simulink model "ASSIG2_v3"  (R2020a)
settings: Solver=FixedStepAuto  StartTime=0.0  StopTime=10.0  FixedStep=1e-3  RelTol=1e-3  EnableMultiTasking=on
undefined symbols (not defined in the file): A0, A1, D0, D1, D10, D11, D12, D13, D2, D3, D4, D5, D6, D7, D8, D9, magnitude, PTA0, PTA1, PTA2, PTB2, PTB23, PTB3, PTB9, PTC16, PTC17, PTC2, PTC3, PTC4, PTD0, PTD1, PTD2, PTD3
libraries: frdmk64flib x19, etargetslib x2
settings Model: ExtModeTrigDuration=5  Creator=Nour  LastModifiedBy=Khaled
settings OptimizationCC: EnhancedBackFolding=on  PassReuseOutputArgsAs=Individual arguments  ZeroExternalMemoryAtStartup=off  ZeroInternalMemoryAtStartup=off  MaxStackSize=64  OptimizeBlockOrder=speed  DifferentSizesBufferReuse=on  OptimizationCustomize=off  EfficientTunableParamExpr=on
settings DebuggingCC: ParameterTunabilityLossMsg=error
settings HardwareCC: ProdBitPerPointer=32  ProdBitPerSizeT=32  ProdBitPerPtrDiffT=32  ProdLargestAtomicInteger=Long  ProdLargestAtomicFloat=Double  ProdWordSize=32  ProdHWDeviceType=ARM Compatible->ARM Cortex
settings SFSimCC: MATLABDynamicMemAlloc=off
settings RTWCC: SystemTargetFile=ert.tlc  HardwareBoard=NXP FRDM-K64F  TemplateMakefile=ert_default_tmf  Toolchain=GNU Tools for ARM Embedded Processors
settings CodeAppCC: ForceParamTrailComments=on  IgnoreCustomStorageClasses=off  OperatorAnnotations=on  SimulinkDataObjDesc=on  SFDataObjDesc=on  InsertBlockDesc=on

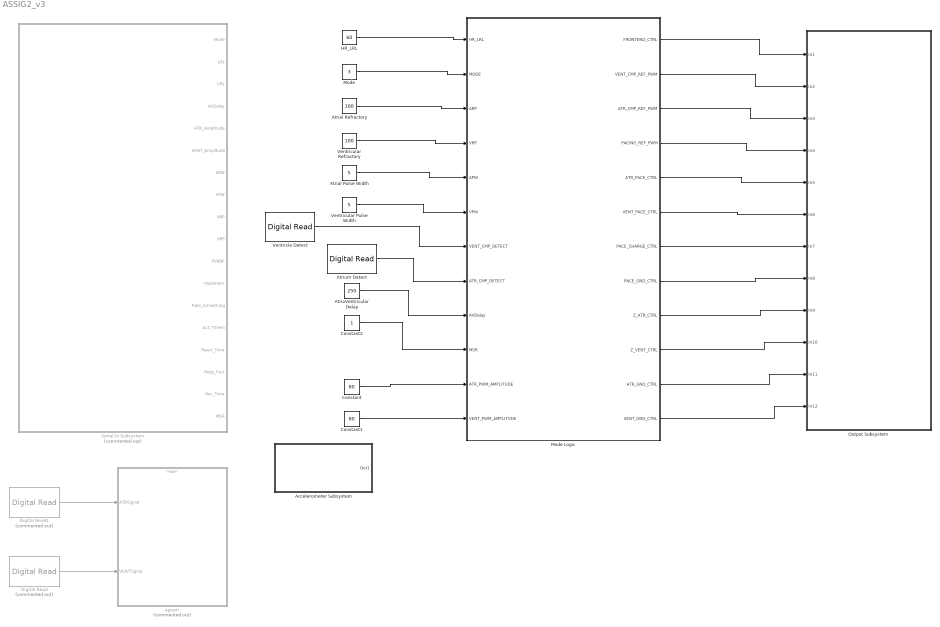
== system ASSIG2_v3 ==
  Accelerometer Subsystem : Subsystem
  Atrial Pulse Width : Constant  Value=5  OutDataTypeStr=uint16
  Atrial Refractory : Constant  Value=100  OutDataTypeStr=uint16
  AtrioVentricular Delay : Constant  Value=250  OutDataTypeStr=uint16
  Atrium Detect : frdmk64flib/Digital Read  Whichpin=PTC16 (D0)  SampleTime=-1
  Constant : Constant  Value=80  OutDataTypeStr=uint16
  Constant1 : Constant  Value=80  OutDataTypeStr=uint16
  Constant2 : Constant  OutDataTypeStr=uint16
  Digital Read : frdmk64flib/Digital Read  Commented=on  Whichpin=PTB3 (A1)  SampleTime=-1
  Digital Read1 : frdmk64flib/Digital Read  Commented=on  Whichpin=PTB2 (A0)  SampleTime=-1
  HR_LRL : Constant  Value=60  OutDataTypeStr=uint16
  Mode : Constant  Value=3  OutDataTypeStr=uint16
  Mode Logic : Stateflow chart  TreatAsAtomicUnit=on
  Output Subsystem : Subsystem
  Serial In Subsystem : Subsystem  Commented=on
  Ventricle Detect : frdmk64flib/Digital Read  Whichpin=PTC17 (D1)  SampleTime=-1
  Ventricular Pulse Width : Constant  Value=5  OutDataTypeStr=uint16
  Ventricular Refractory : Constant  Value=100  OutDataTypeStr=uint16
  egram : Subsystem  Commented=on
  wires:
  HR_LRL/1 -> Mode Logic/1(HR_LRL)
  Mode/1 -> Mode Logic/2(MODE)
  Atrial Refractory/1 -> Mode Logic/3(ARP)
  Ventricular Refractory/1 -> Mode Logic/4(VRP)
  Atrial Pulse Width/1 -> Mode Logic/5(APW)
  Ventricle Detect/1 -> Mode Logic/7(VENT_CMP_DETECT)
  Atrium Detect/1 -> Mode Logic/8(ATR_CMP_DETECT)
  Ventricular Pulse Width/1 -> Mode Logic/6(VPW)
  AtrioVentricular Delay/1 -> Mode Logic/9(AVDelay)
  Constant2/1 -> Mode Logic/10(MSR)
  Constant/1 -> Mode Logic/11(ATR_PWM_AMPLITUDE)
  Constant1/1 -> Mode Logic/12(VENT_PWM_AMPLITUDE)
  Mode Logic/1(FRONTEND_CTRL) -> Output Subsystem/1(In1)
  Mode Logic/2(VENT_CMP_REF_PWM) -> Output Subsystem/2(In2)
  Mode Logic/3(ATR_CMP_REF_PWM) -> Output Subsystem/3(In3)
  Mode Logic/4(PACING_REF_PWM) -> Output Subsystem/4(In4)
  Mode Logic/5(ATR_PACE_CTRL) -> Output Subsystem/5(In5)
  Mode Logic/6(VENT_PACE_CTRL) -> Output Subsystem/6(In6)
  Mode Logic/7(PACE_CHARGE_CTRL) -> Output Subsystem/7(In7)
  Mode Logic/8(PACE_GND_CTRL) -> Output Subsystem/8(In8)
  Mode Logic/9(Z_ATR_CTRL) -> Output Subsystem/9(In9)
  Mode Logic/10(Z_VENT_CTRL) -> Output Subsystem/10(In10)
  Mode Logic/11(ATR_GND_CTRL) -> Output Subsystem/11(In11)
  Mode Logic/12(VENT_GND_CTRL) -> Output Subsystem/12(In12)
  Digital Read/1 -> egram/2(VENTSignal)
  Digital Read1/1 -> egram/1(ATRSignal)

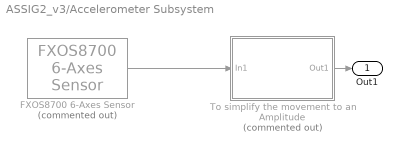
== system ASSIG2_v3/Accelerometer Subsystem ==
  FXOS8700 6-Axes Sensor : frdmk64flib/FXOS8700 6-Axes Sensor  Commented=on  Activesensor=Accelerometer only  ODR=800Hz  HybridODR=400Hz  Accelfullrange=-4g to +4g  SampleTime=-1
  To simplify the movement to an Amplitude : Subsystem  Commented=on
  Out1 : Outport
  wires:
  FXOS8700 6-Axes Sensor/1 -> To simplify the movement to an Amplitude/1(In1)
  To simplify the movement to an Amplitude/1(Out1) -> Out1/1

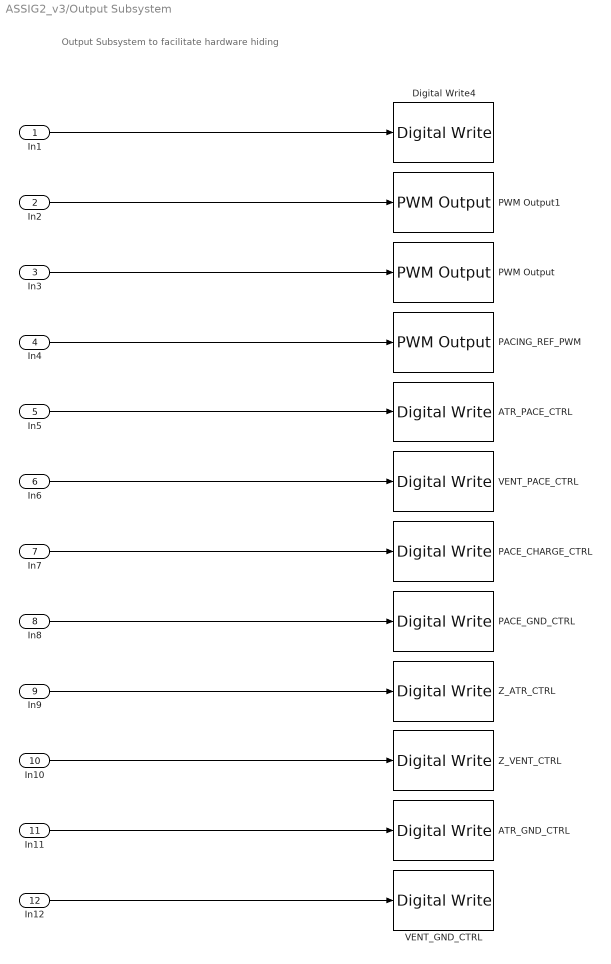
== system ASSIG2_v3/Output Subsystem ==
  note: Output Subsystem to facilitate hardware hiding
  In1 : Inport
  In2 : Inport  Port=2
  In3 : Inport  Port=3
  In4 : Inport  Port=4
  In5 : Inport  Port=5
  In6 : Inport  Port=6
  In7 : Inport  Port=7
  In8 : Inport  Port=8
  In9 : Inport  Port=9
  In10 : Inport  Port=10
  In11 : Inport  Port=11
  In12 : Inport  Port=12
  ATR_GND_CTRL : frdmk64flib/Digital Write  Whichpin=PTD2 (D11)
  ATR_PACE_CTRL : frdmk64flib/Digital Write  Whichpin=PTA0 (D8)
  Digital Write4 : frdmk64flib/Digital Write  Whichpin=PTD1 (D13)
  PACE_CHARGE_CTRL : frdmk64flib/Digital Write  Whichpin=PTB9 (D2)
  PACE_GND_CTRL : frdmk64flib/Digital Write  Whichpin=PTD0 (D10)
  PACING_REF_PWM : frdmk64flib/PWM Output  Whichpin=PTA2 (D5)  InitialFrequency=2000  InitialDutyCycle=80
  PWM Output : frdmk64flib/PWM Output  Whichpin=PTC2 (D6)  InitialFrequency=2000  InitialDutyCycle=20
  PWM Output1 : frdmk64flib/PWM Output  Whichpin=PTA1 (D3)  InitialFrequency=2000  InitialDutyCycle=20
  VENT_GND_CTRL : frdmk64flib/Digital Write  Whichpin=PTD3 (D12)
  VENT_PACE_CTRL : frdmk64flib/Digital Write  Whichpin=PTC4 (D9)
  Z_ATR_CTRL : frdmk64flib/Digital Write  Whichpin=PTB23 (D4)
  Z_VENT_CTRL : frdmk64flib/Digital Write  Whichpin=PTC3 (D7)
  wires:
  In7/1 -> PACE_CHARGE_CTRL/1
  In12/1 -> VENT_GND_CTRL/1
  In1/1 -> Digital Write4/1
  In4/1 -> PACING_REF_PWM/1
  In8/1 -> PACE_GND_CTRL/1
  In6/1 -> VENT_PACE_CTRL/1
  In9/1 -> Z_ATR_CTRL/1
  In10/1 -> Z_VENT_CTRL/1
  In11/1 -> ATR_GND_CTRL/1
  In2/1 -> PWM Output1/1
  In5/1 -> ATR_PACE_CTRL/1
  In3/1 -> PWM Output/1

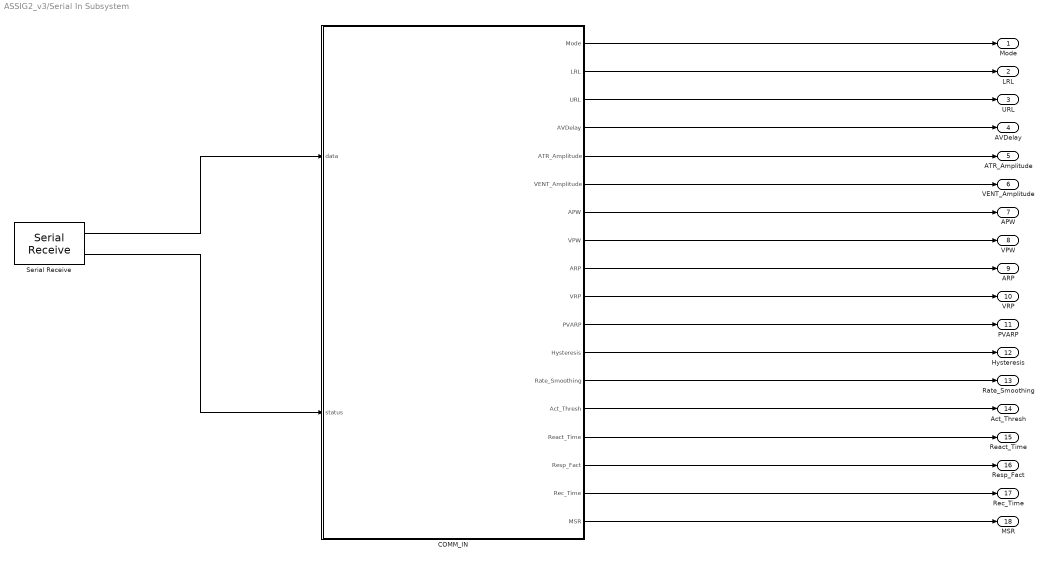
== system ASSIG2_v3/Serial In Subsystem ==
  COMM_IN : Stateflow chart  TreatAsAtomicUnit=on
  Serial Receive : frdmk64flib/Serial Receive  SCIModule=0  Baudrate=uint32(9600)  Parity=None  StopBits=1  HardwareFlowControl=None  ByteOrder=LittleEndian  DataType=uint8  DataLength=24  BlockingMode=off  OutputStatus=on  SampleTime=-1
  Mode : Outport
  LRL : Outport  Port=2
  URL : Outport  Port=3
  AVDelay : Outport  Port=4
  ATR_Amplitude : Outport  Port=5
  VENT_Amplitude : Outport  Port=6
  APW : Outport  Port=7
  VPW : Outport  Port=8
  ARP : Outport  Port=9
  VRP : Outport  Port=10
  PVARP : Outport  Port=11
  Hysteresis : Outport  Port=12
  Rate_Smoothing : Outport  Port=13
  Act_Thresh : Outport  Port=14
  React_Time : Outport  Port=15
  Resp_Fact : Outport  Port=16
  Rec_Time : Outport  Port=17
  MSR : Outport  Port=18
  wires:
  COMM_IN/3(URL) -> URL/1
  COMM_IN/9(ARP) -> ARP/1
  COMM_IN/4(AVDelay) -> AVDelay/1
  Serial Receive/1 -> COMM_IN/1(data)
  COMM_IN/2(LRL) -> LRL/1
  COMM_IN/8(VPW) -> VPW/1
  Serial Receive/2 -> COMM_IN/2(status)
  COMM_IN/6(VENT_Amplitude) -> VENT_Amplitude/1
  COMM_IN/5(ATR_Amplitude) -> ATR_Amplitude/1
  COMM_IN/16(Resp_Fact) -> Resp_Fact/1
  COMM_IN/1(Mode) -> Mode/1
  COMM_IN/13(Rate_Smoothing) -> Rate_Smoothing/1
  COMM_IN/15(React_Time) -> React_Time/1
  COMM_IN/10(VRP) -> VRP/1
  COMM_IN/7(APW) -> APW/1
  COMM_IN/17(Rec_Time) -> Rec_Time/1
  COMM_IN/18(MSR) -> MSR/1
  COMM_IN/12(Hysteresis) -> Hysteresis/1
  COMM_IN/14(Act_Thresh) -> Act_Thresh/1
  COMM_IN/11(PVARP) -> PVARP/1

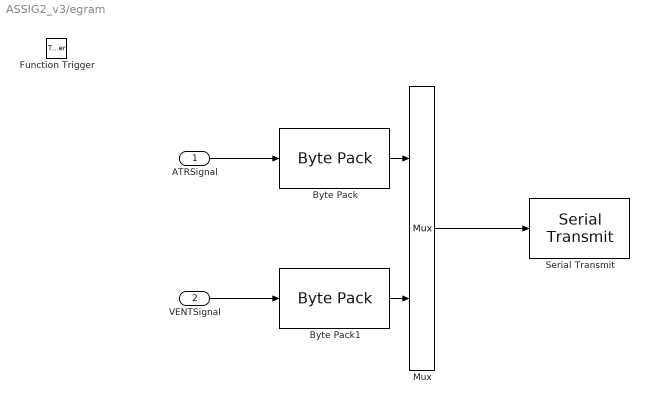
== system ASSIG2_v3/egram ==
  ATRSignal : Inport
  VENTSignal : Inport  Port=2
  Function Trigger : TriggerPort  TriggerType=function-call  IsSimulinkFunction=on  FunctionName=send_params  VariantControl=Variant  PortDimensions=1
  Byte Pack : etargetslib/Byte Pack  datatypes={'double'}  byteAlign=1
  Byte Pack1 : etargetslib/Byte Pack  datatypes={'double'}  byteAlign=1
  Mux : Mux  Inputs=2
  Serial Transmit : frdmk64flib/Serial Transmit  SCIModule=0  Baudrate=uint32(9600)  Parity=None  StopBits=1  HardwareFlowControl=None  ByteOrder=LittleEndian  BlockingMode=on  OutputStatus=off
  wires:
  ATRSignal/1 -> Byte Pack/1
  Byte Pack1/1 -> Mux/2
  Byte Pack/1 -> Mux/1
  VENTSignal/1 -> Byte Pack1/1
  Mux/1 -> Serial Transmit/1

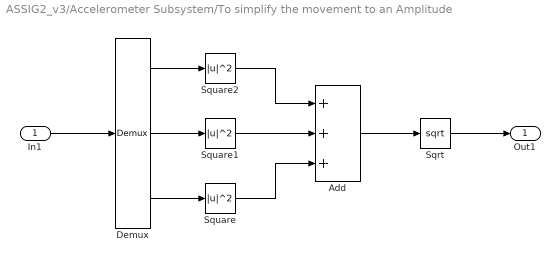
== system ASSIG2_v3/Accelerometer Subsystem/To simplify the movement to an Amplitude ==
  In1 : Inport
  Add : Sum  Inputs=+++
  Demux : Demux  Outputs=3
  Sqrt : Sqrt  OutputSignalType=real  OutDataTypeStr=uint16  SaturateOnIntegerOverflow=on
  Square : Math  Operator=magnitude^2  SaturateOnIntegerOverflow=on
  Square1 : Math  Operator=magnitude^2  SaturateOnIntegerOverflow=on
  Square2 : Math  Operator=magnitude^2  SaturateOnIntegerOverflow=on
  Out1 : Outport
  wires:
  In1/1 -> Demux/1
  Demux/3 -> Square/1
  Demux/2 -> Square1/1
  Demux/1 -> Square2/1
  Square2/1 -> Add/1
  Square1/1 -> Add/2
  Square/1 -> Add/3
  Add/1 -> Sqrt/1
  Sqrt/1 -> Out1/1

== stateflow chart ASSIG2_v3/Serial In Subsystem/COMM_IN ==
  state SET_PARAM
    %% setting parameter values through
    %% serial communication
    Mode = typecast(data(3), 'uint8');
    URL = typecast(data(4), 'uint8');
    LRL = typecast(data(5), 'uint8');
    VENT_Amplitude = typecast(data(6), 'uint8');
    VPW = typecast(data(7), 'uint8');
    ATR_Amplitude = typecast(data(8), 'uint8');
    APW = typecast(data(9), 'uint8');
    VRP = typecast(data(10:11), 'uint16');
    ARP = typecast(data(12:13), 'uint16');
    PVARP = typecast(data(14:15), 'uint16');
    Hysteresis = typecast(data(16), 'uint8');
    Rate_Smoothing = typecast(data(17), 'uint8');
    AVDelay = typecast(data(18: 19), 'uint16');
    MSR = typecast(data(20), 'uint8');
    Act_Thresh = typecast(data(21), 'uint8');
    React_Time = typecast(data(22), 'uint8');
    Resp_Fact = typecast(data(23), 'uint8');
    Rec_Time = typecast(data(24), 'uint8');
  state INITIAL
    %% Setting initial, default values of parameters
    entry:
    Mode = 0;
    URL = 0;
    LRL = 0;
    VENT_Amplitude = 0;
    VPW = 0;
    ATR_Amplitude = 0;
    APW = 0;
    VRP = 0;
    ARP = 0;
    PVARP = 0;
    Hysteresis = 0;
    Rate_Smoothing = 0;
    AVDelay = 0;
    MSR = 0;
    Act_Thresh = 0;
    React_Time = 0;
    Resp_Fact = 0;
    Rec_Time = 0;
  state STANDBY
    %% Waiting for COM
  state ECHO_PARAM
    entry:
    %%send_params();
    %% returnparams();
  (junction 15) -> SET_PARAM [order 2] : [data(2) == hex2dec('55')]
  SET_PARAM -> STANDBY
  (default) -> INITIAL
  (junction 13) -> STANDBY [order 2]
  INITIAL -> STANDBY
  STANDBY -> (junction 13) : [status == 0]
  (junction 13) -> (junction 15) [order 1] : [data(1) == hex2dec('16')]
  (junction 15) -> ECHO_PARAM [order 1] : [data(2) == hex2dec('22')]
  ECHO_PARAM -> STANDBY
  data: data input uint8 size=[24;1]; status input uint8 size=[1;1]; Mode output uint8; LRL output uint8; URL output uint8; AVDelay output uint16; ATR_Amplitude output uint8; VENT_Amplitude output uint8; APW output uint8; VPW output uint8; ARP output uint16; VRP output uint16; PVARP output uint16; Hysteresis output uint8; Rate_Smoothing output uint8; Act_Thresh output uint8; React_Time output uint8; Resp_Fact output uint8; Rec_Time output uint8; MSR output uint8

== stateflow chart ASSIG2_v3/Mode Logic ==
  state AOOR [commented out]
  state VOOR [commented out]
  state DOOR [commented out]
  state Entry
    %% MODE Values:
    %% 1: AOO
    %% 2: VOO
    %% 3: AAI
    %% 4: VVI
    %% 5: DOO
    %% 6: AOOR
    %% 7: VOOR
    %% 8: AAIR
    %% 9:  VVIR
    %% 10: DOOR
    entry:
    ATR_CMP_REF_PWM = 80;
    VENT_CMP_REF_PWM = 20;
    %% FRONTEND_CTRL = false;
    delay = 0;
  state AAI
    state Charge
      entry:
      ATR_PACE_CTRL = false;
      VENT_PACE_CTRL = false;
      PACING_REF_PWM = ATR_PWM_AMPLITUDE;
      PACE_CHARGE_CTRL = true;
      %Discharging Blocking Capacitor
      PACE_GND_CTRL = true;
      VENT_PACE_CTRL = false;
      Z_ATR_CTRL = false;
      Z_VENT_CTRL = false;
      %% ATR_PACE_CTRL = false;
      ATR_GND_CTRL = true;
      VENT_GND_CTRL = false;FRONTEND_CTRL = true;
    state Pace
      entry:
      PACE_CHARGE_CTRL = false;
      PACE_GND_CTRL = true;
      ATR_PACE_CTRL = true;
      ATR_GND_CTRL = false;
      Z_ATR_CTRL = false;
      Z_VENT_CTRL = false;
      VENT_GND_CTRL = false;
      VENT_PACE_CTRL = false;
      %% FRONTEND_CTRL = true;
    state Refractor
      entry:
      ATR_PACE_CTRL = false;
      VENT_PACE_CTRL = false;
      PACING_REF_PWM = ATR_PWM_AMPLITUDE;
      PACE_CHARGE_CTRL = true;
      %Discharging Blocking Capacitor
      PACE_GND_CTRL = true;
      VENT_PACE_CTRL = false;
      Z_ATR_CTRL = false;
      Z_VENT_CTRL = false;
      %% ATR_PACE_CTRL = false;
      ATR_GND_CTRL = true;
      VENT_GND_CTRL = false;
      %% FRONTEND_CTRL = true;
    (default) -> AAI.Charge
    AAI.Charge -> AAI.Pace [order 1] : [after((60000 / HR_LRL - ARP - delay), msec)]
    AAI.Charge -> AAI.Refractor [order 2] : [ATR_CMP_DETECT == true]{delay = 0}
    AAI.Refractor -> AAI.Charge : [after(ARP, msec)]
    AAI.Pace -> AAI.Refractor : [after(APW, msec)]{delay = APW}
  state AAIR [commented out]
  state VVI
    state Charge
      %% Charge C22, Discharge C21
      entry:
      ATR_PACE_CTRL = false;
      VENT_PACE_CTRL = false;
      PACING_REF_PWM = VENT_PWM_AMPLITUDE;
      PACE_CHARGE_CTRL = true;
      %Dishcharging Blocking Capacitor
      PACE_GND_CTRL = true;
      Z_ATR_CTRL = false;
      Z_VENT_CTRL = false;
      ATR_GND_CTRL = false;
      VENT_GND_CTRL = true;
      FRONTEND_CTRL = true;
    state Pace
      entry:
      PACE_CHARGE_CTRL = false;
      PACE_GND_CTRL = true;
      ATR_PACE_CTRL = false;
      ATR_GND_CTRL = false;
      Z_ATR_CTRL = false;
      Z_VENT_CTRL = false;
      VENT_GND_CTRL = false;
      VENT_PACE_CTRL = true;
      %% FRONTEND_CTRL = true;
    state Refractor
      %% Charge C22, Discharge C21
      entry:
      ATR_PACE_CTRL = false;
      VENT_PACE_CTRL = false;
      PACING_REF_PWM = VENT_PWM_AMPLITUDE;
      PACE_CHARGE_CTRL = true;
      %Dishcharging Blocking Capacitor
      PACE_GND_CTRL = true;
      Z_ATR_CTRL = false;
      Z_VENT_CTRL = false;
      ATR_GND_CTRL = false;
      VENT_GND_CTRL = true;
      %% FRONTEND_CTRL = true;
    (default) -> VVI.Charge
    VVI.Charge -> VVI.Pace [order 1] : [after((60000 / HR_LRL - VRP - delay), msec)]
    VVI.Charge -> VVI.Refractor [order 2] : [VENT_CMP_DETECT == true]{delay = 0}
    VVI.Refractor -> VVI.Charge : [after(VRP, msec)]
    VVI.Pace -> VVI.Refractor : [after(VPW, msec)]{delay = VPW}
  state VVIR [commented out]
  state DOO
    state ATRCharge
      entry:
      ATR_PACE_CTRL = false;
      VENT_PACE_CTRL = false;
      PACING_REF_PWM = ATR_PWM_AMPLITUDE;
      PACE_CHARGE_CTRL = true;
      %Discharging Blocking Capacitor
      PACE_GND_CTRL = true;
      VENT_PACE_CTRL = false;
      Z_ATR_CTRL = false;
      Z_VENT_CTRL = false;
      %% ATR_PACE_CTRL = false;
      ATR_GND_CTRL = true;
      VENT_GND_CTRL = false;
    state ATRPace
      entry:
      entry:
      PACE_CHARGE_CTRL = false;
      PACE_GND_CTRL = true;
      ATR_PACE_CTRL = true;
      ATR_GND_CTRL = false;
      Z_ATR_CTRL = false;
      Z_VENT_CTRL = false;
      VENT_GND_CTRL = false;
      VENT_PACE_CTRL = false;
    state VentPace
      entry:
      PACE_CHARGE_CTRL = false;
      PACE_GND_CTRL = true;
      ATR_PACE_CTRL = false;
      ATR_GND_CTRL = false;
      Z_ATR_CTRL = false;
      Z_VENT_CTRL = false;
      VENT_GND_CTRL = false;
      VENT_PACE_CTRL = true;
    state VENTCharge
      %% Charge C22, Discharge C21
      entry:
      ATR_PACE_CTRL = false;
      VENT_PACE_CTRL = false;
      PACING_REF_PWM = VENT_PWM_AMPLITUDE;
      PACE_CHARGE_CTRL = true;
      %Dishcharging Blocking Capacitor
      PACE_GND_CTRL = true;
      Z_ATR_CTRL = false;
      Z_VENT_CTRL = false;
      ATR_GND_CTRL = false;
      VENT_GND_CTRL = true;
    (default) -> ATRCharge
    ATRCharge -> ATRPace : [after((60000 / HR_LRL - AVDelay - APW - VPW), msec)]
    VentPace -> ATRCharge : [after(VPW, msec)]
    ATRPace -> VENTCharge : [after(APW, msec)]
    VENTCharge -> VentPace : [after(AVDelay, msec)]
  state AOO
    state CHARGE
      entry:
      ATR_PACE_CTRL = false;
      VENT_PACE_CTRL = false;
      PACING_REF_PWM = ATR_PWM_AMPLITUDE;
      PACE_CHARGE_CTRL = true;
      %Discharging Blocking Capacitor
      PACE_GND_CTRL = true;
      VENT_PACE_CTRL = false;
      Z_ATR_CTRL = false;
      Z_VENT_CTRL = false;
      %% ATR_PACE_CTRL = false;
      ATR_GND_CTRL = true;
      VENT_GND_CTRL = false;
    state PACE
      entry:
      PACE_CHARGE_CTRL = false;
      PACE_GND_CTRL = true;
      ATR_PACE_CTRL = true;
      ATR_GND_CTRL = false;
      Z_ATR_CTRL = false;
      Z_VENT_CTRL = false;
      VENT_GND_CTRL = false;
      VENT_PACE_CTRL = false;
    (default) -> AOO.PACE
    AOO.PACE -> AOO.CHARGE : [after(APW, msec)]
    AOO.CHARGE -> AOO.PACE : [after((60000 / HR_LRL - APW), msec)]
  state VOO
    state PACE
      entry:
      PACE_CHARGE_CTRL = false;
      PACE_GND_CTRL = true;
      ATR_PACE_CTRL = false;
      ATR_GND_CTRL = false;
      Z_ATR_CTRL = false;
      Z_VENT_CTRL = false;
      VENT_GND_CTRL = false;
      VENT_PACE_CTRL = true;
    state CHARGE
      %% Charge C22, Discharge C21
      entry:
      ATR_PACE_CTRL = false;
      VENT_PACE_CTRL = false;
      PACING_REF_PWM = VENT_PWM_AMPLITUDE;
      PACE_CHARGE_CTRL = true;
      %Dishcharging Blocking Capacitor
      PACE_GND_CTRL = true;
      Z_ATR_CTRL = false;
      Z_VENT_CTRL = false;
      ATR_GND_CTRL = false;
      VENT_GND_CTRL = true;
    (default) -> VOO.PACE
    VOO.PACE -> VOO.CHARGE : [after(VPW, msec)]
    VOO.CHARGE -> VOO.PACE : [after((60000 / HR_LRL - VPW), msec)]
  Entry -> DOOR [commented out] : [MODE == 10]
  Entry -> AOOR [commented out] : [MODE == 6]
  Entry -> VOOR [commented out] : [MODE == 7]
  (default) -> Entry
  Entry -> AAI [order 4] : [MODE == 3]
  Entry -> AAIR [commented out] : [MODE == 8]
  Entry -> VVI [order 5] : [MODE == 4]
  Entry -> VVIR [commented out] : [MODE == 9]
  Entry -> AOO [order 1] : [MODE == 1]
  Entry -> VOO [order 2] : [MODE == 2]
  Entry -> DOO [order 3] : [MODE == 5]
  data: FRONTEND_CTRL output boolean; delay local uint16; HR_LRL input uint16; MODE input uint16; VENT_CMP_REF_PWM output uint16; ATR_CMP_REF_PWM output uint16; ARP input uint16; VRP input uint16; APW input uint16; VPW input uint16; VENT_CMP_DETECT input boolean; ATR_CMP_DETECT input boolean; AVDelay input uint16; MSR input uint16; ATR_PWM_AMPLITUDE input uint16; VENT_PWM_AMPLITUDE input uint16; PACING_REF_PWM output uint16; ATR_PACE_CTRL output boolean; VENT_PACE_CTRL output boolean; PACE_CHARGE_CTRL output boolean; PACE_GND_CTRL output boolean; Z_ATR_CTRL output boolean; Z_VENT_CTRL output boolean; ATR_GND_CTRL output boolean; VENT_GND_CTRL output boolean
